simulink model "practice10"  (Simulink 7.9)
settings: Solver=ode45  StartTime=0.0  StopTime=10.0  RelTol=1e-3
settings Model: Creator=sony  LastModifiedBy=sony

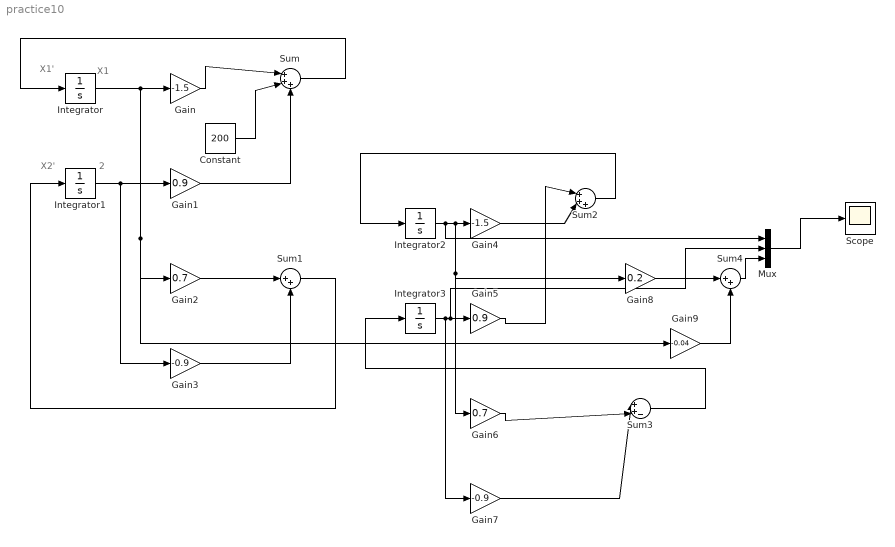
== system practice10 ==
  note: X1'
  note: X1
  note: X2'
  note: 2
  Constant : Constant  Value=200
  Gain : Gain  Gain=-1.5
  Gain1 : Gain  Gain=0.9
  Gain2 : Gain  Gain=0.7
  Gain3 : Gain  Gain=-0.9
  Gain4 : Gain  Gain=-1.5
  Gain5 : Gain  Gain=0.9
  Gain6 : Gain  Gain=0.7
  Gain7 : Gain  Gain=-0.9
  Gain8 : Gain  Gain=0.2
  Gain9 : Gain  Gain=-0.04
  Integrator{,1..3} (4 alike) : Integrator
  Mux : Mux  Inputs=3
  Scope : Scope
  Sum : Sum  Inputs=|+++
  Sum1 : Sum  Inputs=|++
  Sum2 : Sum  Inputs=|+++
  Sum3 : Sum  Inputs=|++-
  Sum4 : Sum  Inputs=|++
  wires:
  Integrator/1 -> Gain/1, Gain2/1, Gain9/1
  Integrator1/1 -> Gain1/1, Gain3/1
  Gain/1 -> Sum/1
  Constant/1 -> Sum/2
  Gain1/1 -> Sum/3
  Sum/1 -> Integrator/1
  Gain2/1 -> Sum1/1
  Gain3/1 -> Sum1/2
  Sum1/1 -> Integrator1/1
  Integrator2/1 -> Gain4/1, Gain6/1, Gain8/1, Mux/1
  Integrator3/1 -> Gain7/1, Gain5/1, Mux/2
  Gain4/1 -> Sum2/2
  Sum2/1 -> Integrator2/1
  Gain6/1 -> Sum3/2
  Sum3/1 -> Integrator3/1
  Mux/1 -> Scope/1
  Gain5/1 -> Sum2/1
  Gain7/1 -> Sum3/1
  Gain9/1 -> Sum4/2
  Gain8/1 -> Sum4/1
  Sum4/1 -> Mux/3
